simulink model "sampleModel1502"  (R2023a)
settings: Solver=VariableStepAuto  StartTime=0.0  StopTime=10.0  RelTol=1e-3
libraries: hdlsllib x5, simulink x1
settings Model: Creator=user1  LastModifiedBy=user1

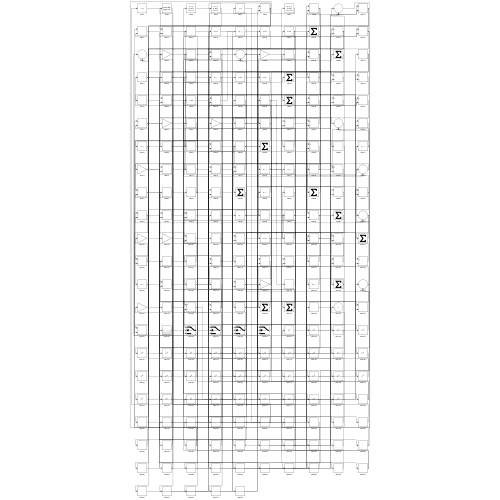
[thumbnail: Simulink's stored preview of the top-level diagram]
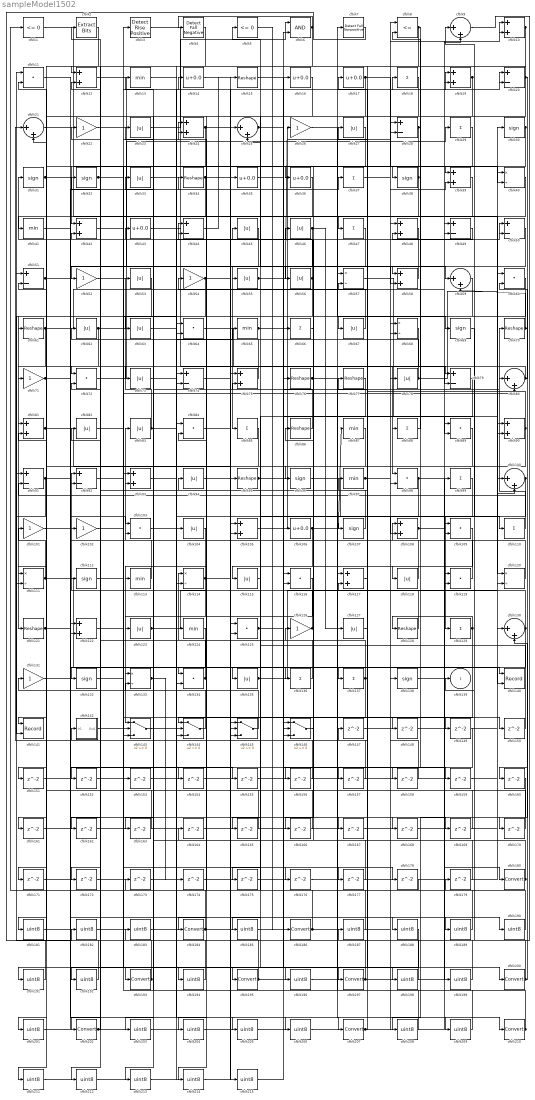
== system sampleModel1502 ==
  cfblk1 : hdlsllib/Logic and Bit Operations/Compare To Zero  relop=<=  OutDataTypeStr=boolean
  cfblk{10,12,19,24,39,42,48,58,75,81,90,93,105,108,117,122} (16 alike) : Sum
  cfblk{9,21,25,59,80,100,130} (7 alike) : Sum  Inputs=|++
  cfblk{22,26,52,54,71,101..102,126,131} (9 alike) : Gain
  cfblk{11,60,64,72,84,89,98,103,109,116,119,125,134} (13 alike) : DotProduct  OutDataTypeStr=Inherit: Inherit via internal rule
  cfblk{23,27,33,45..46,53,55..56,62..63,67,73,78,82..83,94,104,115,118,123,127,135} (22 alike) : Abs  SaturateOnIntegerOverflow=off
  cfblk{14,16..17,35..36,43,106} (7 alike) : Bias  Bias=0.0  SaturateOnIntegerOverflow=off
  cfblk{30..32,38,69,96,107,112,132,138} (10 alike) : Signum
  cfblk{18,29,37,47,66,85,88,99,110,129,136..137} (12 alike) : Sum  Inputs=+
  cfblk{40,57,68,111,114,120,133} (7 alike) : Product  Inputs=*/  RndMeth=Zero  SaturateOnIntegerOverflow=on
  cfblk{13,41,65,87,97,113,124} (7 alike) : MinMax
  cfblk{15,34,61,70,76..77,86,95,121,128} (10 alike) : Reshape
  cfblk140 : Record  FileSettingsInternal="{\"entries\":[{\"content\":{\"excelSettings\":{\"content\":{},\"type\":\"Streamout.ExcelSettings\"}},\"type\":\"Streamout.FileSettingStorage\",\"uuid\":\"\"}],\"packageUris\":[\"http:\\/\\/schema.mathworks.com\\/mf0\\/streamout_blocks\\/R2020a\"],\"version\":\"1.0\"}"  Layout=[1 1]  SignalsInternal="{\"entries\":[{\"content\":{\"signals\":[{\"content\":{\"blockPath\":[],\"dimensions\":[1],\"domain\":\"\",\"lineColor\":\"#a2142f\",\"plots\":[1],\"port\":1,\"signalID\":1298,\"signalName\":\"XY Graph:1\"},\"type\":\"RecordBlkView.Signal\",\"uuid\":\"\"},{\"content\":{\"blockPath\":[],\"dimensions\":[1],\"domain\":\"\",\"lineColor\":\"#139fff\",\"plots\":[1],\"port\":2,\"signalID\":1301,\"signalName\":\"XY Graph:2\"},\"type\":\"RecordBlkView.Signal\",\"uuid\":\"\"}]},\"type\":\"RecordBlkView.InputSignals\",\"uuid\":\"\"}],\"packageUris\":[\"http:\\/\\/schema.mathworks.com\\/mf0\\/streamout_blocks\\/R2020a\"],\"version\":\"1.0\"}"  VisualizationBindings="{\"xyplotplugin\":{\"info\":[{\"series\":[{\"bindingParametersList\":[{\"parameter\":\"X-Axis\",\"signalID\":1298,\"signalName\":\"XY Graph:1\"},{\"parameter\":\"Y-Axis\",\"signalID\":1301,\"signalName\":\"XY Graph:2\"}],\"seriesID\":63275}],\"subplotID\":1}]}}"  CompatibilityTag=XY  st=-1
  cfblk141 : Record  FileSettingsInternal="{\"entries\":[{\"content\":{\"excelSettings\":{\"content\":{},\"type\":\"Streamout.ExcelSettings\"}},\"type\":\"Streamout.FileSettingStorage\",\"uuid\":\"\"}],\"packageUris\":[\"http:\\/\\/schema.mathworks.com\\/mf0\\/streamout_blocks\\/R2020a\"],\"version\":\"1.0\"}"  Layout=[1 1]  SignalsInternal="{\"entries\":[{\"content\":{\"signals\":[{\"content\":{\"blockPath\":[],\"dimensions\":[1],\"domain\":\"\",\"lineColor\":\"#a2142f\",\"plots\":[1],\"port\":1,\"signalID\":1306,\"signalName\":\"XY Graph:1\"},\"type\":\"RecordBlkView.Signal\",\"uuid\":\"\"},{\"content\":{\"blockPath\":[],\"dimensions\":[1],\"domain\":\"\",\"lineColor\":\"#139fff\",\"plots\":[1],\"port\":2,\"signalID\":1309,\"signalName\":\"XY Graph:2\"},\"type\":\"RecordBlkView.Signal\",\"uuid\":\"\"}]},\"type\":\"RecordBlkView.InputSignals\",\"uuid\":\"\"}],\"packageUris\":[\"http:\\/\\/schema.mathworks.com\\/mf0\\/streamout_blocks\\/R2020a\"],\"version\":\"1.0\"}"  VisualizationBindings="{\"xyplotplugin\":{\"info\":[{\"series\":[{\"bindingParametersList\":[{\"parameter\":\"X-Axis\",\"signalID\":1306,\"signalName\":\"XY Graph:1\"},{\"parameter\":\"Y-Axis\",\"signalID\":1309,\"signalName\":\"XY Graph:2\"}],\"seriesID\":32852}],\"subplotID\":1}]}}"  CompatibilityTag=XY  st=-1
  cfblk142 : Subsystem
      settings: LibrarySourceBlock=|
      | hdlsllib/Ports &
      | Subsystems/Subsystem
  cfblk{143..146} (4 alike) : Switch  SaturateOnIntegerOverflow=off  InputSameDT=off
  cfblk{147..179} (33 alike) : Delay  SampleTime=1
  cfblk{180,184,186,193,195,197,200,202,207,210} (10 alike) : DataTypeConversion  SaturateOnIntegerOverflow=off  RndMeth=Floor
  cfblk{181..183,185,187..192,194,196,198..199,201,203..206,208..209,211..215} (26 alike) : DataTypeConversion  OutDataTypeStr=uint8  SaturateOnIntegerOverflow=off  RndMeth=Floor
  cfblk2 : simulink/Logic and Bit Operations/Extract Bits  bitsToExtract=Upper half  numBits=8  bitIdxRange=[0 7]  outScalingMode=Preserve fixed-point scaling
      settings: LibrarySourceBlock=|
      | hdlsllib/Logic and Bit
      | Operations/Extract Bits
  cfblk{20,28,44,49..51,74,79,91..92} (10 alike) : Sum  Inputs=+-
  cfblk3 : hdlsllib/Logic and Bit Operations/Detect Rise Positive  vinit=0  OutDataTypeStr=boolean
  cfblk4 : hdlsllib/Logic and Bit Operations/Detect Fall Negative  vinit=0  OutDataTypeStr=boolean
  cfblk5 : hdlsllib/Logic and Bit Operations/Compare To Zero  relop=<=  OutDataTypeStr=boolean
  cfblk6 : Logic  AllPortsSameDT=off  OutDataTypeStr=boolean
  cfblk7 : hdlsllib/Logic and Bit Operations/Detect Fall Nonpositive  vinit=0  OutDataTypeStr=boolean
  cfblk8 : RelationalOperator  Operator=<=  OutDataTypeStr=boolean  InputSameDT=off
  cfblk139 : Outport  VectorParamsAs1DForOutWhenUnconnected=off
  wires:
  cfblk95/1 -> cfblk50/1, cfblk159/1
  cfblk44/1 -> cfblk15/1
  cfblk66/1 -> cfblk132/1
  cfblk104/1 -> cfblk143/1
  cfblk106/1 -> cfblk87/1, cfblk146/3
  cfblk123/1 -> cfblk31/1, cfblk50/2
  cfblk45/1 -> cfblk85/1
  cfblk133/1 -> cfblk21/1, cfblk174/1
  cfblk23/1 -> cfblk6/1
  cfblk126/1 -> cfblk92/1, cfblk46/1
  cfblk134/1 -> cfblk114/1, cfblk33/1
  cfblk79/1 -> cfblk144/1
  cfblk28/1 -> cfblk125/2, cfblk41/1, cfblk148/1
  cfblk118/1 -> cfblk83/1
  cfblk111/1 -> cfblk133/1, cfblk101/1
  cfblk13/1 -> cfblk114/2
  cfblk74/1 -> cfblk210/1
  cfblk100/1 -> cfblk91/2, cfblk185/1
  cfblk84/1 -> cfblk107/1
  cfblk52/1 -> cfblk29/1
  cfblk30/1 -> cfblk42/1, cfblk134/2
  cfblk22/1 -> cfblk59/1
  cfblk77/1 -> cfblk115/1
  cfblk124/1 -> cfblk202/1
  cfblk21/1 -> cfblk120/1
  cfblk138/1 -> cfblk180/1
  cfblk10/1 -> cfblk118/1, cfblk71/1
  cfblk55/1 -> cfblk26/1, cfblk88/1
  cfblk110/1 -> cfblk70/1
  cfblk78/1 -> cfblk30/1, cfblk13/1
  cfblk113/1 -> cfblk92/2
  cfblk32/1 -> cfblk176/1, cfblk177/1
  cfblk94/1 -> cfblk35/1
  cfblk130/1 -> cfblk84/2, cfblk134/1
  cfblk40/1 -> cfblk123/1
  cfblk81/1 -> cfblk105/1, cfblk205/1
  cfblk114/1 -> cfblk113/1, cfblk20/2, cfblk163/1
  cfblk105/1 -> cfblk8/1
  cfblk97/1 -> cfblk77/1, cfblk39/2
  cfblk62/1 -> cfblk37/1, cfblk80/2, cfblk111/1
  cfblk144/1 -> cfblk43/1
  cfblk12/1 -> cfblk38/1
  cfblk125/1 -> cfblk80/1, cfblk198/1
  cfblk54/1 -> cfblk121/1, cfblk168/1
  cfblk38/1 -> cfblk36/1, cfblk162/1
  cfblk5/1 -> cfblk186/1
  cfblk33/1 -> cfblk98/1
  cfblk96/1 -> cfblk129/1
  cfblk103/1 -> cfblk19/1
  cfblk75/1 -> cfblk32/1
  cfblk120/1 -> cfblk108/1
  cfblk90/1 -> cfblk27/1, cfblk137/1
  cfblk71/1 -> cfblk154/1, cfblk155/1
  cfblk91/1 -> cfblk140/1, cfblk141/2
  cfblk56/1 -> cfblk44/1, cfblk111/2
  cfblk35/1 -> cfblk106/1
  cfblk128/1 -> cfblk45/1
  cfblk131/1 -> cfblk193/1
  cfblk136/1 -> cfblk82/1
  cfblk64/1 -> cfblk79/1
  cfblk27/1 -> cfblk56/1
  cfblk117/1 -> cfblk197/1
  cfblk67/1 -> cfblk54/1
  cfblk3/1 -> cfblk100/1
  cfblk31/1 -> cfblk103/1, cfblk58/2
  cfblk42/1 -> cfblk64/2
  cfblk49/1 -> cfblk48/2
  cfblk48/1 -> cfblk96/1
  cfblk69/1 -> cfblk109/1
  cfblk98/1 -> cfblk135/1, cfblk110/1
  cfblk73/1 -> cfblk109/2
  cfblk51/1 -> cfblk122/2, cfblk206/1
  cfblk36/1 -> cfblk141/1
  cfblk1/1 -> cfblk40/2
  cfblk24/1 -> cfblk25/1, cfblk143/3
  cfblk129/1 -> cfblk128/1, cfblk145/2
  cfblk86/1 -> cfblk23/1
  cfblk137/1 -> cfblk17/1, cfblk62/1, cfblk75/2, cfblk214/1
  cfblk112/1 -> cfblk3/1
  cfblk127/1 -> cfblk97/1
  cfblk58/1 -> cfblk52/1
  cfblk34/1 -> cfblk108/2, cfblk63/1
  cfblk43/1 -> cfblk66/1
  cfblk19/1 -> cfblk21/2, cfblk201/1
  cfblk20/1 -> cfblk12/1, cfblk160/1, cfblk161/1
  cfblk16/1 -> cfblk184/1
  cfblk18/1 -> cfblk144/2
  cfblk8/1 -> cfblk47/1, cfblk58/1
  cfblk99/1 -> cfblk195/1
  cfblk6/1 -> cfblk4/1, cfblk61/1, cfblk172/1, cfblk192/1
  cfblk57/1 -> cfblk89/2
  cfblk122/1 -> cfblk24/1
  cfblk93/1 -> cfblk207/1
  cfblk102/1 -> cfblk200/1
  cfblk83/1 -> cfblk53/1, cfblk136/1
  cfblk76/1 -> cfblk18/1, cfblk209/1
  cfblk143/1 -> cfblk65/1
  cfblk135/1 -> cfblk60/1, cfblk169/1
  cfblk145/1 -> cfblk51/2
  cfblk119/1 -> cfblk44/2
  cfblk108/1 -> cfblk9/2, cfblk150/1
  cfblk72/1 -> cfblk20/1
  cfblk15/1 -> cfblk140/2
  cfblk101/1 -> cfblk34/1
  cfblk25/1 -> cfblk90/2, cfblk178/1
  cfblk92/1 -> cfblk14/1
  cfblk26/1 -> cfblk69/1
  cfblk121/1 -> cfblk167/1, cfblk181/1
  cfblk65/1 -> cfblk76/1, cfblk79/2
  cfblk4/1 -> cfblk144/3
  cfblk46/1 -> cfblk105/2, cfblk127/1
  cfblk88/1 -> cfblk8/2
  cfblk17/1 -> cfblk73/1, cfblk55/1, cfblk39/1
  cfblk37/1 -> cfblk10/1
  cfblk61/1 -> cfblk10/2, cfblk81/1
  cfblk107/1 -> cfblk2/1
  cfblk60/1 -> cfblk67/1
  cfblk146/1 -> cfblk86/1
  cfblk80/1 -> cfblk72/1, cfblk60/2
  cfblk70/1 -> cfblk59/2, cfblk170/1
  cfblk147/1 -> cfblk40/1
  cfblk148/1 -> cfblk89/1
  cfblk132/1 -> cfblk149/1
  cfblk150/1 -> cfblk25/2
  cfblk87/1 -> cfblk151/1
  cfblk151/1 -> cfblk122/1
  cfblk53/1 -> cfblk152/1
  cfblk152/1 -> cfblk125/1
  cfblk82/1 -> cfblk153/1
  cfblk153/1 -> cfblk120/2
  cfblk154/1 -> cfblk146/1
  cfblk155/1 -> cfblk19/2
  cfblk47/1 -> cfblk156/1
  cfblk156/1 -> cfblk84/1
  cfblk29/1 -> cfblk157/1
  cfblk157/1 -> cfblk51/1
  cfblk50/1 -> cfblk158/1
  cfblk158/1 -> cfblk48/1
  cfblk159/1 -> cfblk9/1
  cfblk161/1 -> cfblk6/2
  cfblk162/1 -> cfblk12/2
  cfblk163/1 -> cfblk81/2
  cfblk164/1 -> cfblk28/1
  cfblk115/1 -> cfblk165/1
  cfblk165/1 -> cfblk133/2
  cfblk39/1 -> cfblk166/1
  cfblk166/1 -> cfblk143/2
  cfblk167/1 -> cfblk100/2
  cfblk169/1 -> cfblk57/2
  cfblk170/1 -> cfblk24/2
  cfblk59/1 -> cfblk171/1
  cfblk171/1 -> cfblk146/2
  cfblk172/1 -> cfblk49/2
  cfblk173/1 -> cfblk145/3
  cfblk174/1 -> cfblk145/1
  cfblk109/1 -> cfblk175/1
  cfblk175/1 -> cfblk130/1
  cfblk176/1 -> cfblk90/1
  cfblk177/1 -> cfblk75/1
  cfblk178/1 -> cfblk1/1
  cfblk179/1 -> cfblk103/2
  cfblk180/1 -> cfblk164/1, cfblk126/1
  cfblk181/1 -> cfblk138/1
  cfblk7/1 -> cfblk182/1
  cfblk182/1 -> cfblk104/1
  cfblk9/1 -> cfblk183/1
  cfblk183/1 -> cfblk7/1
  cfblk184/1 -> cfblk72/2, cfblk28/2
  cfblk185/1 -> cfblk16/1
  cfblk186/1 -> cfblk173/1, cfblk94/1
  cfblk187/1 -> cfblk5/1
  cfblk142/1(Out1) -> cfblk188/1
  cfblk63/1 -> cfblk189/1
  cfblk189/1 -> cfblk142/1(In1)
  cfblk11/1 -> cfblk190/1
  cfblk190/1 -> cfblk139/1
  cfblk188/1 -> cfblk191/1
  cfblk191/1 -> cfblk11/1
  cfblk192/1 -> cfblk11/2
  cfblk193/1 -> cfblk22/1, cfblk112/1
  cfblk89/1 -> cfblk194/1
  cfblk194/1 -> cfblk131/1
  cfblk195/1 -> cfblk98/2, cfblk91/1
  cfblk41/1 -> cfblk196/1
  cfblk196/1 -> cfblk99/1
  cfblk197/1 -> cfblk49/1, cfblk64/1
  cfblk198/1 -> cfblk117/1
  cfblk168/1 -> cfblk199/1
  cfblk199/1 -> cfblk117/2
  cfblk200/1 -> cfblk179/1, cfblk130/2
  cfblk201/1 -> cfblk102/1
  cfblk202/1 -> cfblk119/2, cfblk42/2
  cfblk85/1 -> cfblk203/1
  cfblk203/1 -> cfblk124/1
  cfblk68/1 -> cfblk204/1
  cfblk204/1 -> cfblk78/1
  cfblk205/1 -> cfblk68/1
  cfblk206/1 -> cfblk68/2
  cfblk207/1 -> cfblk187/1, cfblk119/1
  cfblk160/1 -> cfblk208/1
  cfblk208/1 -> cfblk93/1
  cfblk209/1 -> cfblk93/2
  cfblk210/1 -> cfblk147/1, cfblk57/1
  cfblk2/1 -> cfblk211/1
  cfblk211/1 -> cfblk74/1
  cfblk149/1 -> cfblk212/1
  cfblk212/1 -> cfblk74/2
  cfblk116/1 -> cfblk213/1
  cfblk213/1 -> cfblk95/1
  cfblk214/1 -> cfblk116/1
  cfblk14/1 -> cfblk215/1
  cfblk215/1 -> cfblk116/2

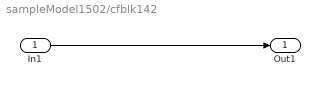
== system sampleModel1502/cfblk142 ==
  In1 : Inport
  Out1 : Outport
  wires:
  In1/1 -> Out1/1
